simulink model "rover_unreal_cosim"  (R2024b)
settings: Solver=FixedStepAuto  StartTime=0.0  StopTime=inf  FixedStep=0.02  RelTol=1e-3
InitFcn:
  | addpath('/home/dinuk/Desktop/project/Rover-Room-SIM/matlab'); setup_ros_humble();
StartFcn:
  | simulink_teleop_start();
StopFcn:
  | simulink_teleop_stop();
undefined symbols (not defined in the file): angular, linear, simulink_teleop_ang, simulink_teleop_lin
libraries: ros2lib x3, sim3dlib x1, sim3dautolib x1
settings Model: Creator=dinuk  LastModifiedBy=dinuk

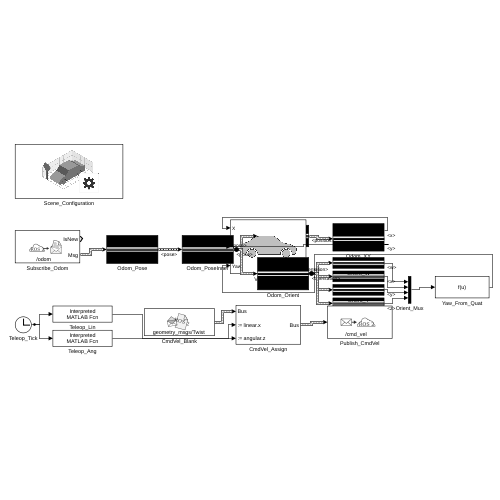
[thumbnail: Simulink's stored preview of the top-level diagram]
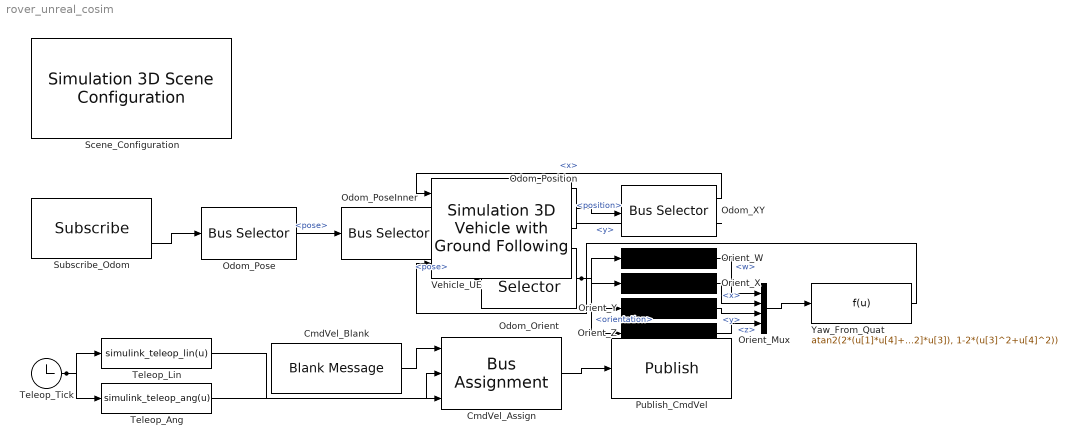
== system rover_unreal_cosim ==
  CmdVel_Assign : BusAssignment  AssignedSignals=linear.x,angular.z
  CmdVel_Blank : ros2lib/Blank Message  messageClass=Message  entityType=geometry_msgs/Twist  messageType=geometry_msgs/Twist  SampleTime=0.02
      link override Constant: OutDataTypeStr=Bus: SL_Bus_geometry_msgs_Twist
  Odom_Orient : BusSelector  OutputSignals=orientation
  Odom_Pose : BusSelector  OutputSignals=pose
  Odom_PoseInner : BusSelector  OutputSignals=pose
  Odom_Position : BusSelector  OutputSignals=position
  Odom_XY : BusSelector  OutputSignals=x,y
  Orient_Mux : Mux
  Orient_W : BusSelector  OutputSignals=w
  Orient_X : BusSelector  OutputSignals=x
  Orient_Y : BusSelector  OutputSignals=y
  Orient_Z : BusSelector  OutputSignals=z
  Publish_CmdVel : ros2lib/Publish  topicSource=Specify your own  topic=/cmd_vel  messageType=geometry_msgs/Twist  QOSHistory=Keep last  QOSDepth=10  QOSReliability=Reliable  QOSDurability=Volatile  QOSDeadline=Inf  QOSLifespan=Inf  QOSLiveliness=Automatic  QOSLeaseDuration=Inf  QOSAvoidROSNamespaceConventions=off
      link override SignalSpecification: OutDataTypeStr=Bus: SL_Bus_geometry_msgs_Twist
      link override SinkBlock: ROSTopic=/cmd_vel  ROSMessageType=geometry_msgs/Twist  SLBusName=SL_Bus_geometry_msgs_Twist  ModelName=rover_unreal_cosim  BlockId=Pub_rover_unreal_cosim_20
  Scene_Configuration : sim3dlib/Simulation 3D Scene Configuration  Priority=0  ProjectFormat=Unreal Editor  SceneDesc=Straight road  ProjectName=/home/dinuk/MATLAB/R2024b/toolbox/shared/sim3d_projects/automotive_project_linux/UE/LinuxNoEditor/VehicleSimulation.sh  ScenePath=/Game/Maps/MyRoom  UEProjPath=/home/dinuk/Desktop/project/Rover-Room-SIM/RoverSIMUunreal-Linux/RoverTwin/RoverTwin.uproject  EnableOpenDRIVE=off  vehTagList={'Scene Origin'}  vehTag=Scene Origin  FreeCameraInitialTranslation=[0, 0, 0]  FreeCameraDefaultInitialTranslation=[-6, 0, 2]  FreeCameraInitialRotation=[0, 0, 0]  FreeCameraDefaultInitialRotation=[0, -15, 0]  OpVisEn=off  Ts=0.02  EnableWindow=on  EnableRemoteAccess=off  EnableWeather=off  SunAzimuth=90  SunAltitude=40.0  EnableGeospatialSun=off  Latitude=0  Longitude=0  Date=2023-01-01  Time=10:30:00  GeoTimeZone=-5.0  SunDaylightSaving=off  wind=1  clouds=10  EnableVolumetricClouds=off  CloudCoverage=0  CloudAltitude=6  fog=0  rain=0  RaindropsEffect=off  SnowDensity=0  EnableGeospatial=off  UseTrueOrigin=off  OriginHeight=200  OriginLatitude=40.744652  OriginLongitude=-73.988864  MapStyle=Aerial  AdditionalAssetIDs=[]  UseAdvancedSunSky=off  SolarTime=11  TimeZone=-5  Day=21  Month=9  Year=2022  UseDaylightSavingTime=on  DSTStartDay=10  DSTStartMonth=3  DSTEndDay=3  DSTEndMonth=11  DSTSwitchHour=2  sensorTag=MainCamera1  sensorId=1  sensorName=MainCamera1  mountLoc=Origin  offsetFlag=off  tmountOffset=[0, 0, 0]  rmountOffset=[0, 0, 0]  HorizontalResolution=1280  VerticalResolution=720  HorizontalFOV=60  mountPoint=[0 0 0]  mountOrientation=[0 0 0]  aMode=aMode  ID=1  GeoTrigger=Inactive
  Subscribe_Odom : ros2lib/Subscribe  topicSource=Specify your own  topic=/odom  messageType=nav_msgs/Odometry  sampleTime=0.02  QOSHistory=Keep last  QOSDepth=10  QOSReliability=Reliable  QOSDurability=Volatile  QOSDeadline=Inf  QOSLifespan=Inf  QOSLiveliness=Automatic  QOSLeaseDuration=Inf  QOSAvoidROSNamespaceConventions=off
      link override Constant: OutDataTypeStr=Bus: SL_Bus_nav_msgs_Odometry
      link override SourceBlock: ROSTopic=/odom  ROSMessageType=nav_msgs/Odometry  SLBusName=SL_Bus_nav_msgs_Odometry  ModelName=rover_unreal_cosim  BlockId=Sub_rover_unreal_cosim_2
  Teleop_Ang : MATLABFcn  MATLABFcn=simulink_teleop_ang(u)
  Teleop_Lin : MATLABFcn  MATLABFcn=simulink_teleop_lin(u)
  Teleop_Tick : Clock
  Vehicle_UE : sim3dautolib/Simulation 3D Vehicle with Ground Following  Priority=-1  PassVehMesh=Muscle car  MeshPath=/MathWorksAutomotiveContent/Vehicles/SmallCar/Meshes/SK_SmallCar.SK_SmallCar  TrackWidth=0.28  WheelBase=0.22  WheelRadius=0.05  VehColor=Blue  InitialPos=[0, 0, 0]  InitialRot=[0, 0, 0]  ActorName=SimulinkVehicle1  SampleTime=-1  ActorType=SimulinkVehicle  ID=1  aMode=3  ActorTag=SimulinkVehicle1  CoordinateScheme=ISO  VehLightsControl=off  HeadlightColor=[ 1, 1, 1 ]  HighBeamIntensity=100000  LowBeamIntensity=60000  HighBeamConeAngle=70  LowBeamConeAngle=70  LeftHeadlightOrientation=[ 0, 0 ]  RightHeadlightOrientation=[ 0, 0 ]  BrakelightIntensity=500  ReverselightIntensity=500  SignallightIntensity=500  SignallightPeriod=1  SignalPulseWidth=50  TransformOutportEnabled=off
      settings: LibrarySourceBlock=drivingsim3d/Simulation 3D Vehicle with Ground Following
  Yaw_From_Quat : Fcn  Expr=atan2(2*(u[1]*u[4]+u[2]*u[3]), 1-2*(u[3]^2+u[4]^2))
  wires:
  Teleop_Tick/1 -> Teleop_Lin/1, Teleop_Ang/1
  CmdVel_Blank/1 -> CmdVel_Assign/1
  Teleop_Lin/1 -> CmdVel_Assign/2
  Teleop_Ang/1 -> CmdVel_Assign/3
  CmdVel_Assign/1 -> Publish_CmdVel/1
  Subscribe_Odom/2 -> Odom_Pose/1
  Odom_Pose/1 -> Odom_PoseInner/1  "<pose>"
  Odom_PoseInner/1 -> Odom_Position/1, Odom_Orient/1  "<pose>"
  Odom_Position/1 -> Odom_XY/1  "<position>"
  Odom_Orient/1 -> Orient_W/1, Orient_X/1, Orient_Y/1, Orient_Z/1  "<orientation>"
  Orient_W/1 -> Orient_Mux/1  "<w>"
  Orient_X/1 -> Orient_Mux/2  "<x>"
  Orient_Y/1 -> Orient_Mux/3  "<y>"
  Orient_Z/1 -> Orient_Mux/4  "<z>"
  Orient_Mux/1 -> Yaw_From_Quat/1
  Odom_XY/1 -> Vehicle_UE/1  "<x>"
  Odom_XY/2 -> Vehicle_UE/2  "<y>"
  Yaw_From_Quat/1 -> Vehicle_UE/3
